simulink model "cpu_von_nuemann"  (R2020a)
settings: Solver=VariableStepAuto  StartTime=0.0  StopTime=10.0  RelTol=1e-3
libraries: simulink_extras x402, msbPllFoundation x1
(part 7 of 64)

== system cpu_von_nuemann/CPU/ALU/Multiplier/Subsystem7/Subsystem4 ==
  In1 : Inport
  In2 : Inport  Port=2
  In3 : Inport  Port=3
  In4 : Inport  Port=4
  In5 : Inport  Port=5
  In6 : Inport  Port=6
  In7 : Inport  Port=7
  In8 : Inport  Port=8
  In9 : Inport  Port=9
  In10 : Inport  Port=10
  In11 : Inport  Port=11
  In12 : Inport  Port=12
  In13 : Inport  Port=13
  In14 : Inport  Port=14
  In15 : Inport  Port=15
  In16 : Inport  Port=16
  Constant16 : Constant  Value=0
  Constant17 : Constant  Value=0
  Display{16..19} (4 alike) : Display
  Logical Operator : Logic  Operator=XOR  AllPortsSameDT=off  OutDataTypeStr=boolean
  Logical Operator1 : Logic  AllPortsSameDT=off  OutDataTypeStr=boolean
  Subsystem1 : Subsystem
  Subsystem15 : Subsystem
  Subsystem2 : Subsystem
  Subsystem3 : Subsystem
  Subsystem4 : Subsystem
  Subsystem5 : Subsystem
  Subsystem6 : Subsystem
  Out1 : Outport
  Out2 : Outport  Port=2
  Out3 : Outport  Port=3
  Out4 : Outport  Port=4
  Out5 : Outport  Port=5
  Out6 : Outport  Port=6
  Out7 : Outport  Port=7
  Out8 : Outport  Port=8
  Out9 : Outport  Port=9
  Out10 : Outport  Port=10
  Out11 : Outport  Port=11
  Out12 : Outport  Port=12
  Out13 : Outport  Port=13
  Out14 : Outport  Port=14
  Out15 : Outport  Port=15
  Out16 : Outport  Port=16
  wires:
  Subsystem3/9(Out9) -> Out16/1
  Subsystem2/6(Out6) -> Subsystem5/13(In13)
  Subsystem5/5(Out5) -> Subsystem4/4(In4)
  Subsystem1/4(Out4) -> Subsystem5/3(In3)
  Subsystem6/1(Out1) -> Display16/1
  Subsystem3/6(Out6) -> Out13/1
  Subsystem2/8(Out8) -> Subsystem5/15(In15)
  In6/1 -> Subsystem3/2(In2), Subsystem2/2(In2)
  Subsystem5/6(Out6) -> Subsystem4/5(In5)
  In4/1 -> Subsystem1/4(In4), Subsystem15/4(In4)
  Subsystem2/2(Out2) -> Subsystem5/9(In9)
  Subsystem2/5(Out5) -> Subsystem5/12(In12)
  Subsystem1/2(Out2) -> Subsystem5/1(In1)
  In2/1 -> Subsystem15/2(In2), Subsystem1/2(In2)
  Subsystem5/8(Out8) -> Subsystem4/7(In7)
  Logical Operator1/1 -> Subsystem6/11(In11)
  Subsystem15/2(Out2) -> Subsystem6/1(In1)
  Subsystem5/3(Out3) -> Subsystem4/2(In2)
  Subsystem2/3(Out3) -> Subsystem5/10(In10)
  Subsystem15/3(Out3) -> Subsystem6/2(In2)
  Constant17/1 -> Subsystem4/11(In11), Subsystem4/10(In10), Subsystem4/9(In9)
  In12/1 -> Subsystem2/8(In8), Subsystem15/8(In8)
  Subsystem4/3(Out3) -> Subsystem6/14(In14)
  Subsystem4/5(Out5) -> Subsystem6/16(In16)
  Subsystem1/6(Out6) -> Subsystem5/5(In5)
  Subsystem2/4(Out4) -> Subsystem5/11(In11)
  Subsystem15/5(Out5) -> Subsystem6/4(In4)
  Subsystem5/1(Out1) -> Logical Operator/1, Logical Operator1/2
  Subsystem1/8(Out8) -> Subsystem5/7(In7)
  Subsystem5/4(Out4) -> Subsystem4/3(In3)
  In8/1 -> Subsystem3/4(In4), Subsystem2/4(In4)
  In10/1 -> Subsystem2/6(In6), Subsystem15/6(In6)
  Subsystem5/2(Out2) -> Subsystem4/1(In1)
  Subsystem6/8(Out8) -> Out7/1
  Constant16/1 -> Subsystem6/10(In10), Subsystem6/9(In9)
  In9/1 -> Subsystem2/5(In5), Subsystem15/5(In5)
  Subsystem1/9(Out9) -> Subsystem5/8(In8)
  Subsystem3/1(Out1) -> Subsystem4/12(In12)
  Subsystem4/9(Out9) -> Out12/1
  In11/1 -> Subsystem2/7(In7), Subsystem15/7(In7)
  In1/1 -> Subsystem1/1(In1), Subsystem15/1(In1)
  In15/1 -> Subsystem3/7(In7), Subsystem1/7(In7)
  Subsystem5/7(Out7) -> Subsystem4/6(In6)
  Subsystem6/3(Out3) -> Out2/1
  In7/1 -> Subsystem3/3(In3), Subsystem2/3(In3)
  Subsystem15/6(Out6) -> Subsystem6/5(In5)
  Subsystem4/8(Out8) -> Out11/1
  Subsystem3/7(Out7) -> Out14/1
  Subsystem15/9(Out9) -> Subsystem6/8(In8)
  Subsystem15/8(Out8) -> Subsystem6/7(In7)
  Subsystem4/7(Out7) -> Out10/1
  Subsystem1/1(Out1) -> Display18/1
  Subsystem6/7(Out7) -> Out6/1
  In16/1 -> Subsystem3/8(In8), Subsystem1/8(In8)
  Subsystem6/4(Out4) -> Out3/1
  In5/1 -> Subsystem3/1(In1), Subsystem2/1(In1)
  Subsystem15/7(Out7) -> Subsystem6/6(In6)
  Subsystem15/4(Out4) -> Subsystem6/3(In3)
  In3/1 -> Subsystem15/3(In3), Subsystem1/3(In3)
  Subsystem3/5(Out5) -> Subsystem4/16(In16)
  Subsystem2/7(Out7) -> Subsystem5/14(In14)
  Logical Operator/1 -> Subsystem6/12(In12)
  Subsystem15/1(Out1) -> Display19/1
  Subsystem6/5(Out5) -> Out4/1
  Subsystem2/1(Out1) -> Display17/1
  Subsystem4/6(Out6) -> Out9/1
  Subsystem5/9(Out9) -> Subsystem4/8(In8)
  Subsystem4/1(Out1) -> Logical Operator/2, Logical Operator1/1
  Subsystem6/9(Out9) -> Out8/1
  Subsystem3/8(Out8) -> Out15/1
  Subsystem4/2(Out2) -> Subsystem6/13(In13)
  Subsystem3/2(Out2) -> Subsystem4/13(In13)
  Subsystem3/4(Out4) -> Subsystem4/15(In15)
  In13/1 -> Subsystem3/5(In5), Subsystem1/5(In5)
  Subsystem4/4(Out4) -> Subsystem6/15(In15)
  Subsystem6/6(Out6) -> Out5/1
  Subsystem2/9(Out9) -> Subsystem5/16(In16)
  Subsystem1/5(Out5) -> Subsystem5/4(In4)
  Subsystem3/3(Out3) -> Subsystem4/14(In14)
  Subsystem6/2(Out2) -> Out1/1
  Subsystem1/7(Out7) -> Subsystem5/6(In6)
  In14/1 -> Subsystem3/6(In6), Subsystem1/6(In6)
  Subsystem1/3(Out3) -> Subsystem5/2(In2)

== system cpu_von_nuemann/CPU/ALU/Multiplier/Subsystem7/Subsystem5 ==
  In1 : Inport
  In2 : Inport  Port=2
  In3 : Inport  Port=3
  In4 : Inport  Port=4
  In5 : Inport  Port=5
  In6 : Inport  Port=6
  In7 : Inport  Port=7
  In8 : Inport  Port=8
  In17 : Inport  Port=9
  In18 : Inport  Port=10
  In19 : Inport  Port=11
  In20 : Inport  Port=12
  14 : Inport  Port=13
  In22 : Inport  Port=14
  In23 : Inport  Port=15
  In24 : Inport  Port=16
  In9 : Inport  Port=17
  In10 : Inport  Port=18
  In11 : Inport  Port=19
  In12 : Inport  Port=20
  In13 : Inport  Port=21
  In14 : Inport  Port=22
  In15 : Inport  Port=23
  In16 : Inport  Port=24
  In25 : Inport  Port=25
  In26 : Inport  Port=26
  In27 : Inport  Port=27
  In28 : Inport  Port=28
  In29 : Inport  Port=29
  In30 : Inport  Port=30
  In31 : Inport  Port=31
  In32 : Inport  Port=32
  Subsystem5 : Subsystem
  Subsystem6 : Subsystem
  Out1 : Outport
  Out2 : Outport  Port=2
  Out3 : Outport  Port=3
  Out4 : Outport  Port=4
  Out5 : Outport  Port=5
  Out6 : Outport  Port=6
  Out7 : Outport  Port=7
  Out8 : Outport  Port=8
  Out9 : Outport  Port=9
  Out10 : Outport  Port=10
  Out11 : Outport  Port=11
  Out12 : Outport  Port=12
  Out13 : Outport  Port=13
  Out14 : Outport  Port=14
  Out15 : Outport  Port=15
  Out16 : Outport  Port=16
  Out17 : Outport  Port=17
  wires:
  In29/1 -> Subsystem6/13(In13)
  In15/1 -> Subsystem5/16(In15)
  In25/1 -> Subsystem6/9(In9)
  Subsystem6/3(Out3) -> Out11/1
  In30/1 -> Subsystem6/14(In14)
  Subsystem6/9(Out9) -> Out17/1
  In32/1 -> Subsystem6/16(In16)
  In18/1 -> Subsystem6/2(In2)
  Subsystem6/6(Out6) -> Out14/1
  In26/1 -> Subsystem6/10(In10)
  Subsystem5/4(Out4) -> Out4/1
  In24/1 -> Subsystem6/8(In8)
  Subsystem5/6(Out6) -> Out6/1
  Subsystem5/1(Out1) -> Out1/1
  In5/1 -> Subsystem5/5(In5)
  In1/1 -> Subsystem5/1(In1)
  In19/1 -> Subsystem6/3(In3)
  Subsystem6/5(Out5) -> Out13/1
  Subsystem5/8(Out8) -> Out8/1
  In28/1 -> Subsystem6/12(In12)
  In10/1 -> Subsystem5/11(In10)
  In14/1 -> Subsystem5/15(In14)
  Subsystem5/3(Out3) -> Out3/1
  In16/1 -> Subsystem5/17(In16)
  Subsystem5/2(Out2) -> Out2/1
  Subsystem5/9(Out9) -> Out9/1
  In8/1 -> Subsystem5/8(In8)
  Subsystem5/5(Out5) -> Out5/1
  In2/1 -> Subsystem5/2(In2)
  In17/1 -> Subsystem6/1(In1)
  In23/1 -> Subsystem6/7(In7)
  Subsystem6/4(Out4) -> Out12/1
  In27/1 -> Subsystem6/11(In11)
  In11/1 -> Subsystem5/12(In11)
  In13/1 -> Subsystem5/14(In13)
  Subsystem6/8(Out8) -> Out16/1
  In22/1 -> Subsystem6/6(In6)
  Subsystem6/1(Out1) -> Subsystem5/9(In17)
  In31/1 -> Subsystem6/15(In15)
  In7/1 -> Subsystem5/7(In7)
  In6/1 -> Subsystem5/6(In6)
  Subsystem6/7(Out7) -> Out15/1
  14/1 -> Subsystem6/5(In5)
  Subsystem6/2(Out2) -> Out10/1
  In4/1 -> Subsystem5/4(In4)
  In20/1 -> Subsystem6/4(In4)
  In12/1 -> Subsystem5/13(In12)
  In3/1 -> Subsystem5/3(In3)
  Subsystem5/7(Out7) -> Out7/1
  In9/1 -> Subsystem5/10(In9)

== system cpu_von_nuemann/CPU/ALU/Multiplier/Subsystem7/Subsystem6 ==
  In1 : Inport
  In2 : Inport  Port=2
  In3 : Inport  Port=3
  In4 : Inport  Port=4
  In5 : Inport  Port=5
  In6 : Inport  Port=6
  In7 : Inport  Port=7
  In8 : Inport  Port=8
  In17 : Inport  Port=9
  In18 : Inport  Port=10
  In19 : Inport  Port=11
  In20 : Inport  Port=12
  14 : Inport  Port=13
  In22 : Inport  Port=14
  In23 : Inport  Port=15
  In24 : Inport  Port=16
  In9 : Inport  Port=17
  In10 : Inport  Port=18
  In11 : Inport  Port=19
  In12 : Inport  Port=20
  In13 : Inport  Port=21
  In14 : Inport  Port=22
  In15 : Inport  Port=23
  In16 : Inport  Port=24
  In25 : Inport  Port=25
  In26 : Inport  Port=26
  In27 : Inport  Port=27
  In28 : Inport  Port=28
  In29 : Inport  Port=29
  In30 : Inport  Port=30
  In31 : Inport  Port=31
  In32 : Inport  Port=32
  Subsystem5 : Subsystem
  Subsystem6 : Subsystem
  Out1 : Outport
  Out2 : Outport  Port=2
  Out3 : Outport  Port=3
  Out4 : Outport  Port=4
  Out5 : Outport  Port=5
  Out6 : Outport  Port=6
  Out7 : Outport  Port=7
  Out8 : Outport  Port=8
  Out9 : Outport  Port=9
  Out10 : Outport  Port=10
  Out11 : Outport  Port=11
  Out12 : Outport  Port=12
  Out13 : Outport  Port=13
  Out14 : Outport  Port=14
  Out15 : Outport  Port=15
  Out16 : Outport  Port=16
  Out17 : Outport  Port=17
  wires:
  In29/1 -> Subsystem6/13(In13)
  In15/1 -> Subsystem5/16(In15)
  In25/1 -> Subsystem6/9(In9)
  Subsystem6/3(Out3) -> Out11/1
  In30/1 -> Subsystem6/14(In14)
  Subsystem6/9(Out9) -> Out17/1
  In32/1 -> Subsystem6/16(In16)
  In18/1 -> Subsystem6/2(In2)
  Subsystem6/6(Out6) -> Out14/1
  In26/1 -> Subsystem6/10(In10)
  Subsystem5/4(Out4) -> Out4/1
  In24/1 -> Subsystem6/8(In8)
  Subsystem5/6(Out6) -> Out6/1
  Subsystem5/1(Out1) -> Out1/1
  In5/1 -> Subsystem5/5(In5)
  In1/1 -> Subsystem5/1(In1)
  In19/1 -> Subsystem6/3(In3)
  Subsystem6/5(Out5) -> Out13/1
  Subsystem5/8(Out8) -> Out8/1
  In28/1 -> Subsystem6/12(In12)
  In10/1 -> Subsystem5/11(In10)
  In14/1 -> Subsystem5/15(In14)
  Subsystem5/3(Out3) -> Out3/1
  In16/1 -> Subsystem5/17(In16)
  Subsystem5/2(Out2) -> Out2/1
  Subsystem5/9(Out9) -> Out9/1
  In8/1 -> Subsystem5/8(In8)
  Subsystem5/5(Out5) -> Out5/1
  In2/1 -> Subsystem5/2(In2)
  In17/1 -> Subsystem6/1(In1)
  In23/1 -> Subsystem6/7(In7)
  Subsystem6/4(Out4) -> Out12/1
  In27/1 -> Subsystem6/11(In11)
  In11/1 -> Subsystem5/12(In11)
  In13/1 -> Subsystem5/14(In13)
  Subsystem6/8(Out8) -> Out16/1
  In22/1 -> Subsystem6/6(In6)
  Subsystem6/1(Out1) -> Subsystem5/9(In17)
  In31/1 -> Subsystem6/15(In15)
  In7/1 -> Subsystem5/7(In7)
  In6/1 -> Subsystem5/6(In6)
  Subsystem6/7(Out7) -> Out15/1
  14/1 -> Subsystem6/5(In5)
  Subsystem6/2(Out2) -> Out10/1
  In4/1 -> Subsystem5/4(In4)
  In20/1 -> Subsystem6/4(In4)
  In12/1 -> Subsystem5/13(In12)
  In3/1 -> Subsystem5/3(In3)
  Subsystem5/7(Out7) -> Out7/1
  In9/1 -> Subsystem5/10(In9)

== system cpu_von_nuemann/CPU/ALU/Subsystem7/Subsystem1/Subsystem1 ==
  In1 : Inport
  In2 : Inport  Port=2
  In3 : Inport  Port=3
  In4 : Inport  Port=4
  In5 : Inport  Port=5
  In7 : Inport  Port=6
  In6 : Inport  Port=7
  Demux{,1..3} (4 alike) : Demux  Outputs=8
  Mux : Mux  Inputs=8
  Subsystem : Subsystem
  Subsystem1 : Subsystem
  Subsystem2 : Subsystem
  Subsystem3 : Subsystem
  Subsystem4 : Subsystem
  Subsystem5 : Subsystem
  Subsystem6 : Subsystem
  Subsystem7 : Subsystem
  Out1 : Outport
  wires:
  Demux3/7 -> Subsystem6/6(In6)
  In6/1 -> Subsystem4/7(In7), Subsystem7/7(In7), Subsystem5/7(In7), Subsystem6/7(In7), Subsystem1/7(In7), Subsystem3/7(In7), Subsystem2/7(In7), Subsystem/7(In7)
  Subsystem3/1(Out1) -> Mux/4
  Demux/1 -> Subsystem/3(In3)
  Demux2/8 -> Subsystem7/5(In5)
  Subsystem1/1(Out1) -> Mux/2
  Subsystem2/1(Out1) -> Mux/3
  Subsystem4/1(Out1) -> Mux/5
  Demux1/2 -> Subsystem1/4(In4)
  Demux/6 -> Subsystem5/3(In3)
  In4/1 -> Demux1/1
  Demux2/7 -> Subsystem6/5(In5)
  In3/1 -> Demux/1
  Demux1/4 -> Subsystem3/4(In4)
  In2/1 -> Subsystem4/2(In2), Subsystem5/2(In2), Subsystem6/2(In2), Subsystem7/2(In2), Subsystem2/2(In2), Subsystem3/2(In2), Subsystem/2(In2), Subsystem1/2(In2)
  Demux3/3 -> Subsystem2/6(In6)
  Subsystem/1(Out1) -> Mux/1
  Subsystem5/1(Out1) -> Mux/6
  In7/1 -> Demux3/1
  Mux/1 -> Out1/1
  Demux/3 -> Subsystem2/3(In3)
  Demux1/8 -> Subsystem7/4(In4)
  Demux3/6 -> Subsystem5/6(In6)
  Demux3/1 -> Subsystem/6(In6)
  Demux3/2 -> Subsystem1/6(In6)
  Subsystem6/1(Out1) -> Mux/7
  Demux1/3 -> Subsystem2/4(In4)
  Demux2/4 -> Subsystem3/5(In5)
  Demux1/5 -> Subsystem4/4(In4)
  In1/1 -> Subsystem6/1(In1), Subsystem7/1(In1), Subsystem4/1(In1), Subsystem5/1(In1), Subsystem2/1(In1), Subsystem3/1(In1), Subsystem/1(In1), Subsystem1/1(In1)
  Demux1/1 -> Subsystem/4(In4)
  Demux3/4 -> Subsystem3/6(In6)
  Demux2/2 -> Subsystem1/5(In5)
  Demux2/6 -> Subsystem5/5(In5)
  Demux/2 -> Subsystem1/3(In3)
  Demux/7 -> Subsystem6/3(In3)
  Demux3/8 -> Subsystem7/6(In6)
  Demux1/6 -> Subsystem5/4(In4)
  Demux/5 -> Subsystem4/3(In3)
  Demux2/5 -> Subsystem4/5(In5)
  Demux/8 -> Subsystem7/3(In3)
  Demux2/3 -> Subsystem2/5(In5)
  Demux3/5 -> Subsystem4/6(In6)
  In5/1 -> Demux2/1
  Demux1/7 -> Subsystem6/4(In4)
  Subsystem7/1(Out1) -> Mux/8
  Demux/4 -> Subsystem3/3(In3)
  Demux2/1 -> Subsystem/5(In5)

== system cpu_von_nuemann/CPU/ALU/Subsystem7/Subsystem1/Subsystem2 ==
  In1 : Inport
  In2 : Inport  Port=2
  In3 : Inport  Port=3
  In4 : Inport  Port=4
  In5 : Inport  Port=5
  In7 : Inport  Port=6
  In6 : Inport  Port=7
  Demux{,1..3} (4 alike) : Demux  Outputs=8
  Mux : Mux  Inputs=8
  Subsystem : Subsystem
  Subsystem1 : Subsystem
  Subsystem2 : Subsystem
  Subsystem3 : Subsystem
  Subsystem4 : Subsystem
  Subsystem5 : Subsystem
  Subsystem6 : Subsystem
  Subsystem7 : Subsystem
  Out1 : Outport
  wires:
  Demux3/7 -> Subsystem6/6(In6)
  In6/1 -> Subsystem4/7(In7), Subsystem7/7(In7), Subsystem5/7(In7), Subsystem6/7(In7), Subsystem1/7(In7), Subsystem3/7(In7), Subsystem2/7(In7), Subsystem/7(In7)
  Subsystem3/1(Out1) -> Mux/4
  Demux/1 -> Subsystem/3(In3)
  Demux2/8 -> Subsystem7/5(In5)
  Subsystem1/1(Out1) -> Mux/2
  Subsystem2/1(Out1) -> Mux/3
  Subsystem4/1(Out1) -> Mux/5
  Demux1/2 -> Subsystem1/4(In4)
  Demux/6 -> Subsystem5/3(In3)
  In4/1 -> Demux1/1
  Demux2/7 -> Subsystem6/5(In5)
  In3/1 -> Demux/1
  Demux1/4 -> Subsystem3/4(In4)
  In2/1 -> Subsystem4/2(In2), Subsystem5/2(In2), Subsystem6/2(In2), Subsystem7/2(In2), Subsystem2/2(In2), Subsystem3/2(In2), Subsystem/2(In2), Subsystem1/2(In2)
  Demux3/3 -> Subsystem2/6(In6)
  Subsystem/1(Out1) -> Mux/1
  Subsystem5/1(Out1) -> Mux/6
  In7/1 -> Demux3/1
  Mux/1 -> Out1/1
  Demux/3 -> Subsystem2/3(In3)
  Demux1/8 -> Subsystem7/4(In4)
  Demux3/6 -> Subsystem5/6(In6)
  Demux3/1 -> Subsystem/6(In6)
  Demux3/2 -> Subsystem1/6(In6)
  Subsystem6/1(Out1) -> Mux/7
  Demux1/3 -> Subsystem2/4(In4)
  Demux2/4 -> Subsystem3/5(In5)
  Demux1/5 -> Subsystem4/4(In4)
  In1/1 -> Subsystem6/1(In1), Subsystem7/1(In1), Subsystem4/1(In1), Subsystem5/1(In1), Subsystem2/1(In1), Subsystem3/1(In1), Subsystem/1(In1), Subsystem1/1(In1)
  Demux1/1 -> Subsystem/4(In4)
  Demux3/4 -> Subsystem3/6(In6)
  Demux2/2 -> Subsystem1/5(In5)
  Demux2/6 -> Subsystem5/5(In5)
  Demux/2 -> Subsystem1/3(In3)
  Demux/7 -> Subsystem6/3(In3)
  Demux3/8 -> Subsystem7/6(In6)
  Demux1/6 -> Subsystem5/4(In4)
  Demux/5 -> Subsystem4/3(In3)
  Demux2/5 -> Subsystem4/5(In5)
  Demux/8 -> Subsystem7/3(In3)
  Demux2/3 -> Subsystem2/5(In5)
  Demux3/5 -> Subsystem4/6(In6)
  In5/1 -> Demux2/1
  Demux1/7 -> Subsystem6/4(In4)
  Subsystem7/1(Out1) -> Mux/8
  Demux/4 -> Subsystem3/3(In3)
  Demux2/1 -> Subsystem/5(In5)

== system cpu_von_nuemann/CPU/ALU/Subsystem7/Subsystem1/Subsystem3 ==
  In1 : Inport
  In2 : Inport  Port=2
  In3 : Inport  Port=3
  In4 : Inport  Port=4
  In5 : Inport  Port=5
  In7 : Inport  Port=6
  In6 : Inport  Port=7
  Demux{,1..3} (4 alike) : Demux  Outputs=8
  Mux : Mux  Inputs=8
  Subsystem : Subsystem
  Subsystem1 : Subsystem
  Subsystem2 : Subsystem
  Subsystem3 : Subsystem
  Subsystem4 : Subsystem
  Subsystem5 : Subsystem
  Subsystem6 : Subsystem
  Subsystem7 : Subsystem
  Out1 : Outport
  wires:
  Demux3/7 -> Subsystem6/6(In6)
  In6/1 -> Subsystem4/7(In7), Subsystem7/7(In7), Subsystem5/7(In7), Subsystem6/7(In7), Subsystem1/7(In7), Subsystem3/7(In7), Subsystem2/7(In7), Subsystem/7(In7)
  Subsystem3/1(Out1) -> Mux/4
  Demux/1 -> Subsystem/3(In3)
  Demux2/8 -> Subsystem7/5(In5)
  Subsystem1/1(Out1) -> Mux/2
  Subsystem2/1(Out1) -> Mux/3
  Subsystem4/1(Out1) -> Mux/5
  Demux1/2 -> Subsystem1/4(In4)
  Demux/6 -> Subsystem5/3(In3)
  In4/1 -> Demux1/1
  Demux2/7 -> Subsystem6/5(In5)
  In3/1 -> Demux/1
  Demux1/4 -> Subsystem3/4(In4)
  In2/1 -> Subsystem4/2(In2), Subsystem5/2(In2), Subsystem6/2(In2), Subsystem7/2(In2), Subsystem2/2(In2), Subsystem3/2(In2), Subsystem/2(In2), Subsystem1/2(In2)
  Demux3/3 -> Subsystem2/6(In6)
  Subsystem/1(Out1) -> Mux/1
  Subsystem5/1(Out1) -> Mux/6
  In7/1 -> Demux3/1
  Mux/1 -> Out1/1
  Demux/3 -> Subsystem2/3(In3)
  Demux1/8 -> Subsystem7/4(In4)
  Demux3/6 -> Subsystem5/6(In6)
  Demux3/1 -> Subsystem/6(In6)
  Demux3/2 -> Subsystem1/6(In6)
  Subsystem6/1(Out1) -> Mux/7
  Demux1/3 -> Subsystem2/4(In4)
  Demux2/4 -> Subsystem3/5(In5)
  Demux1/5 -> Subsystem4/4(In4)
  In1/1 -> Subsystem6/1(In1), Subsystem7/1(In1), Subsystem4/1(In1), Subsystem5/1(In1), Subsystem2/1(In1), Subsystem3/1(In1), Subsystem/1(In1), Subsystem1/1(In1)
  Demux1/1 -> Subsystem/4(In4)
  Demux3/4 -> Subsystem3/6(In6)
  Demux2/2 -> Subsystem1/5(In5)
  Demux2/6 -> Subsystem5/5(In5)
  Demux/2 -> Subsystem1/3(In3)
  Demux/7 -> Subsystem6/3(In3)
  Demux3/8 -> Subsystem7/6(In6)
  Demux1/6 -> Subsystem5/4(In4)
  Demux/5 -> Subsystem4/3(In3)
  Demux2/5 -> Subsystem4/5(In5)
  Demux/8 -> Subsystem7/3(In3)
  Demux2/3 -> Subsystem2/5(In5)
  Demux3/5 -> Subsystem4/6(In6)
  In5/1 -> Demux2/1
  Demux1/7 -> Subsystem6/4(In4)
  Subsystem7/1(Out1) -> Mux/8
  Demux/4 -> Subsystem3/3(In3)
  Demux2/1 -> Subsystem/5(In5)

== system cpu_von_nuemann/CPU/ALU/Subsystem7/Subsystem1/Subsystem4 ==
  In1 : Inport
  In2 : Inport  Port=2
  In3 : Inport  Port=3
  In4 : Inport  Port=4
  In5 : Inport  Port=5
  In7 : Inport  Port=6
  In6 : Inport  Port=7
  Demux{,1..3} (4 alike) : Demux  Outputs=8
  Mux : Mux  Inputs=8
  Subsystem : Subsystem
  Subsystem1 : Subsystem
  Subsystem2 : Subsystem
  Subsystem3 : Subsystem
  Subsystem4 : Subsystem
  Subsystem5 : Subsystem
  Subsystem6 : Subsystem
  Subsystem7 : Subsystem
  Out1 : Outport
  wires:
  Demux3/7 -> Subsystem6/6(In6)
  In6/1 -> Subsystem4/7(In7), Subsystem7/7(In7), Subsystem5/7(In7), Subsystem6/7(In7), Subsystem1/7(In7), Subsystem3/7(In7), Subsystem2/7(In7), Subsystem/7(In7)
  Subsystem3/1(Out1) -> Mux/4
  Demux/1 -> Subsystem/3(In3)
  Demux2/8 -> Subsystem7/5(In5)
  Subsystem1/1(Out1) -> Mux/2
  Subsystem2/1(Out1) -> Mux/3
  Subsystem4/1(Out1) -> Mux/5
  Demux1/2 -> Subsystem1/4(In4)
  Demux/6 -> Subsystem5/3(In3)
  In4/1 -> Demux1/1
  Demux2/7 -> Subsystem6/5(In5)
  In3/1 -> Demux/1
  Demux1/4 -> Subsystem3/4(In4)
  In2/1 -> Subsystem4/2(In2), Subsystem5/2(In2), Subsystem6/2(In2), Subsystem7/2(In2), Subsystem2/2(In2), Subsystem3/2(In2), Subsystem/2(In2), Subsystem1/2(In2)
  Demux3/3 -> Subsystem2/6(In6)
  Subsystem/1(Out1) -> Mux/1
  Subsystem5/1(Out1) -> Mux/6
  In7/1 -> Demux3/1
  Mux/1 -> Out1/1
  Demux/3 -> Subsystem2/3(In3)
  Demux1/8 -> Subsystem7/4(In4)
  Demux3/6 -> Subsystem5/6(In6)
  Demux3/1 -> Subsystem/6(In6)
  Demux3/2 -> Subsystem1/6(In6)
  Subsystem6/1(Out1) -> Mux/7
  Demux1/3 -> Subsystem2/4(In4)
  Demux2/4 -> Subsystem3/5(In5)
  Demux1/5 -> Subsystem4/4(In4)
  In1/1 -> Subsystem6/1(In1), Subsystem7/1(In1), Subsystem4/1(In1), Subsystem5/1(In1), Subsystem2/1(In1), Subsystem3/1(In1), Subsystem/1(In1), Subsystem1/1(In1)
  Demux1/1 -> Subsystem/4(In4)
  Demux3/4 -> Subsystem3/6(In6)
  Demux2/2 -> Subsystem1/5(In5)
  Demux2/6 -> Subsystem5/5(In5)
  Demux/2 -> Subsystem1/3(In3)
  Demux/7 -> Subsystem6/3(In3)
  Demux3/8 -> Subsystem7/6(In6)
  Demux1/6 -> Subsystem5/4(In4)
  Demux/5 -> Subsystem4/3(In3)
  Demux2/5 -> Subsystem4/5(In5)
  Demux/8 -> Subsystem7/3(In3)
  Demux2/3 -> Subsystem2/5(In5)
  Demux3/5 -> Subsystem4/6(In6)
  In5/1 -> Demux2/1
  Demux1/7 -> Subsystem6/4(In4)
  Subsystem7/1(Out1) -> Mux/8
  Demux/4 -> Subsystem3/3(In3)
  Demux2/1 -> Subsystem/5(In5)

== system cpu_von_nuemann/CPU/ALU/Subsystem7/Subsystem1/Subsystem5 ==
  In1 : Inport
  In2 : Inport  Port=2
  In3 : Inport  Port=3
  In4 : Inport  Port=4
  In5 : Inport  Port=5
  In7 : Inport  Port=6
  In6 : Inport  Port=7
  Demux{,1..3} (4 alike) : Demux  Outputs=8
  Mux : Mux  Inputs=8
  Subsystem : Subsystem
  Subsystem1 : Subsystem
  Subsystem2 : Subsystem
  Subsystem3 : Subsystem
  Subsystem4 : Subsystem
  Subsystem5 : Subsystem
  Subsystem6 : Subsystem
  Subsystem7 : Subsystem
  Out1 : Outport
  wires:
  Demux3/7 -> Subsystem6/6(In6)
  In6/1 -> Subsystem4/7(In7), Subsystem7/7(In7), Subsystem5/7(In7), Subsystem6/7(In7), Subsystem1/7(In7), Subsystem3/7(In7), Subsystem2/7(In7), Subsystem/7(In7)
  Subsystem3/1(Out1) -> Mux/4
  Demux/1 -> Subsystem/3(In3)
  Demux2/8 -> Subsystem7/5(In5)
  Subsystem1/1(Out1) -> Mux/2
  Subsystem2/1(Out1) -> Mux/3
  Subsystem4/1(Out1) -> Mux/5
  Demux1/2 -> Subsystem1/4(In4)
  Demux/6 -> Subsystem5/3(In3)
  In4/1 -> Demux1/1
  Demux2/7 -> Subsystem6/5(In5)
  In3/1 -> Demux/1
  Demux1/4 -> Subsystem3/4(In4)
  In2/1 -> Subsystem4/2(In2), Subsystem5/2(In2), Subsystem6/2(In2), Subsystem7/2(In2), Subsystem2/2(In2), Subsystem3/2(In2), Subsystem/2(In2), Subsystem1/2(In2)
  Demux3/3 -> Subsystem2/6(In6)
  Subsystem/1(Out1) -> Mux/1
  Subsystem5/1(Out1) -> Mux/6
  In7/1 -> Demux3/1
  Mux/1 -> Out1/1
  Demux/3 -> Subsystem2/3(In3)
  Demux1/8 -> Subsystem7/4(In4)
  Demux3/6 -> Subsystem5/6(In6)
  Demux3/1 -> Subsystem/6(In6)
  Demux3/2 -> Subsystem1/6(In6)
  Subsystem6/1(Out1) -> Mux/7
  Demux1/3 -> Subsystem2/4(In4)
  Demux2/4 -> Subsystem3/5(In5)
  Demux1/5 -> Subsystem4/4(In4)
  In1/1 -> Subsystem6/1(In1), Subsystem7/1(In1), Subsystem4/1(In1), Subsystem5/1(In1), Subsystem2/1(In1), Subsystem3/1(In1), Subsystem/1(In1), Subsystem1/1(In1)
  Demux1/1 -> Subsystem/4(In4)
  Demux3/4 -> Subsystem3/6(In6)
  Demux2/2 -> Subsystem1/5(In5)
  Demux2/6 -> Subsystem5/5(In5)
  Demux/2 -> Subsystem1/3(In3)
  Demux/7 -> Subsystem6/3(In3)
  Demux3/8 -> Subsystem7/6(In6)
  Demux1/6 -> Subsystem5/4(In4)
  Demux/5 -> Subsystem4/3(In3)
  Demux2/5 -> Subsystem4/5(In5)
  Demux/8 -> Subsystem7/3(In3)
  Demux2/3 -> Subsystem2/5(In5)
  Demux3/5 -> Subsystem4/6(In6)
  In5/1 -> Demux2/1
  Demux1/7 -> Subsystem6/4(In4)
  Subsystem7/1(Out1) -> Mux/8
  Demux/4 -> Subsystem3/3(In3)
  Demux2/1 -> Subsystem/5(In5)

== system cpu_von_nuemann/CPU/ALU/Subsystem7/Subsystem2/Subsystem1 ==
  In1 : Inport
  In2 : Inport  Port=2
  In3 : Inport  Port=3
  In4 : Inport  Port=4
  In5 : Inport  Port=5
  In7 : Inport  Port=6
  In6 : Inport  Port=7
  Demux{,1..3} (4 alike) : Demux  Outputs=8
  Mux : Mux  Inputs=8
  Subsystem : Subsystem
  Subsystem1 : Subsystem
  Subsystem2 : Subsystem
  Subsystem3 : Subsystem
  Subsystem4 : Subsystem
  Subsystem5 : Subsystem
  Subsystem6 : Subsystem
  Subsystem7 : Subsystem
  Out1 : Outport
  wires:
  Demux3/7 -> Subsystem6/6(In6)
  In6/1 -> Subsystem4/7(In7), Subsystem7/7(In7), Subsystem5/7(In7), Subsystem6/7(In7), Subsystem1/7(In7), Subsystem3/7(In7), Subsystem2/7(In7), Subsystem/7(In7)
  Subsystem3/1(Out1) -> Mux/4
  Demux/1 -> Subsystem/3(In3)
  Demux2/8 -> Subsystem7/5(In5)
  Subsystem1/1(Out1) -> Mux/2
  Subsystem2/1(Out1) -> Mux/3
  Subsystem4/1(Out1) -> Mux/5
  Demux1/2 -> Subsystem1/4(In4)
  Demux/6 -> Subsystem5/3(In3)
  In4/1 -> Demux1/1
  Demux2/7 -> Subsystem6/5(In5)
  In3/1 -> Demux/1
  Demux1/4 -> Subsystem3/4(In4)
  In2/1 -> Subsystem4/2(In2), Subsystem5/2(In2), Subsystem6/2(In2), Subsystem7/2(In2), Subsystem2/2(In2), Subsystem3/2(In2), Subsystem/2(In2), Subsystem1/2(In2)
  Demux3/3 -> Subsystem2/6(In6)
  Subsystem/1(Out1) -> Mux/1
  Subsystem5/1(Out1) -> Mux/6
  In7/1 -> Demux3/1
  Mux/1 -> Out1/1
  Demux/3 -> Subsystem2/3(In3)
  Demux1/8 -> Subsystem7/4(In4)
  Demux3/6 -> Subsystem5/6(In6)
  Demux3/1 -> Subsystem/6(In6)
  Demux3/2 -> Subsystem1/6(In6)
  Subsystem6/1(Out1) -> Mux/7
  Demux1/3 -> Subsystem2/4(In4)
  Demux2/4 -> Subsystem3/5(In5)
  Demux1/5 -> Subsystem4/4(In4)
  In1/1 -> Subsystem6/1(In1), Subsystem7/1(In1), Subsystem4/1(In1), Subsystem5/1(In1), Subsystem2/1(In1), Subsystem3/1(In1), Subsystem/1(In1), Subsystem1/1(In1)
  Demux1/1 -> Subsystem/4(In4)
  Demux3/4 -> Subsystem3/6(In6)
  Demux2/2 -> Subsystem1/5(In5)
  Demux2/6 -> Subsystem5/5(In5)
  Demux/2 -> Subsystem1/3(In3)
  Demux/7 -> Subsystem6/3(In3)
  Demux3/8 -> Subsystem7/6(In6)
  Demux1/6 -> Subsystem5/4(In4)
  Demux/5 -> Subsystem4/3(In3)
  Demux2/5 -> Subsystem4/5(In5)
  Demux/8 -> Subsystem7/3(In3)
  Demux2/3 -> Subsystem2/5(In5)
  Demux3/5 -> Subsystem4/6(In6)
  In5/1 -> Demux2/1
  Demux1/7 -> Subsystem6/4(In4)
  Subsystem7/1(Out1) -> Mux/8
  Demux/4 -> Subsystem3/3(In3)
  Demux2/1 -> Subsystem/5(In5)

== system cpu_von_nuemann/CPU/ALU/Subsystem7/Subsystem2/Subsystem2 ==
  In1 : Inport
  In2 : Inport  Port=2
  In3 : Inport  Port=3
  In4 : Inport  Port=4
  In5 : Inport  Port=5
  In7 : Inport  Port=6
  In6 : Inport  Port=7
  Demux{,1..3} (4 alike) : Demux  Outputs=8
  Mux : Mux  Inputs=8
  Subsystem : Subsystem
  Subsystem1 : Subsystem
  Subsystem2 : Subsystem
  Subsystem3 : Subsystem
  Subsystem4 : Subsystem
  Subsystem5 : Subsystem
  Subsystem6 : Subsystem
  Subsystem7 : Subsystem
  Out1 : Outport
  wires:
  Demux3/7 -> Subsystem6/6(In6)
  In6/1 -> Subsystem4/7(In7), Subsystem7/7(In7), Subsystem5/7(In7), Subsystem6/7(In7), Subsystem1/7(In7), Subsystem3/7(In7), Subsystem2/7(In7), Subsystem/7(In7)
  Subsystem3/1(Out1) -> Mux/4
  Demux/1 -> Subsystem/3(In3)
  Demux2/8 -> Subsystem7/5(In5)
  Subsystem1/1(Out1) -> Mux/2
  Subsystem2/1(Out1) -> Mux/3
  Subsystem4/1(Out1) -> Mux/5
  Demux1/2 -> Subsystem1/4(In4)
  Demux/6 -> Subsystem5/3(In3)
  In4/1 -> Demux1/1
  Demux2/7 -> Subsystem6/5(In5)
  In3/1 -> Demux/1
  Demux1/4 -> Subsystem3/4(In4)
  In2/1 -> Subsystem4/2(In2), Subsystem5/2(In2), Subsystem6/2(In2), Subsystem7/2(In2), Subsystem2/2(In2), Subsystem3/2(In2), Subsystem/2(In2), Subsystem1/2(In2)
  Demux3/3 -> Subsystem2/6(In6)
  Subsystem/1(Out1) -> Mux/1
  Subsystem5/1(Out1) -> Mux/6
  In7/1 -> Demux3/1
  Mux/1 -> Out1/1
  Demux/3 -> Subsystem2/3(In3)
  Demux1/8 -> Subsystem7/4(In4)
  Demux3/6 -> Subsystem5/6(In6)
  Demux3/1 -> Subsystem/6(In6)
  Demux3/2 -> Subsystem1/6(In6)
  Subsystem6/1(Out1) -> Mux/7
  Demux1/3 -> Subsystem2/4(In4)
  Demux2/4 -> Subsystem3/5(In5)
  Demux1/5 -> Subsystem4/4(In4)
  In1/1 -> Subsystem6/1(In1), Subsystem7/1(In1), Subsystem4/1(In1), Subsystem5/1(In1), Subsystem2/1(In1), Subsystem3/1(In1), Subsystem/1(In1), Subsystem1/1(In1)
  Demux1/1 -> Subsystem/4(In4)
  Demux3/4 -> Subsystem3/6(In6)
  Demux2/2 -> Subsystem1/5(In5)
  Demux2/6 -> Subsystem5/5(In5)
  Demux/2 -> Subsystem1/3(In3)
  Demux/7 -> Subsystem6/3(In3)
  Demux3/8 -> Subsystem7/6(In6)
  Demux1/6 -> Subsystem5/4(In4)
  Demux/5 -> Subsystem4/3(In3)
  Demux2/5 -> Subsystem4/5(In5)
  Demux/8 -> Subsystem7/3(In3)
  Demux2/3 -> Subsystem2/5(In5)
  Demux3/5 -> Subsystem4/6(In6)
  In5/1 -> Demux2/1
  Demux1/7 -> Subsystem6/4(In4)
  Subsystem7/1(Out1) -> Mux/8
  Demux/4 -> Subsystem3/3(In3)
  Demux2/1 -> Subsystem/5(In5)

== system cpu_von_nuemann/CPU/ALU/Subsystem7/Subsystem2/Subsystem3 ==
  In1 : Inport
  In2 : Inport  Port=2
  In3 : Inport  Port=3
  In4 : Inport  Port=4
  In5 : Inport  Port=5
  In7 : Inport  Port=6
  In6 : Inport  Port=7
  Demux{,1..3} (4 alike) : Demux  Outputs=8
  Mux : Mux  Inputs=8
  Subsystem : Subsystem
  Subsystem1 : Subsystem
  Subsystem2 : Subsystem
  Subsystem3 : Subsystem
  Subsystem4 : Subsystem
  Subsystem5 : Subsystem
  Subsystem6 : Subsystem
  Subsystem7 : Subsystem
  Out1 : Outport
  wires:
  Demux3/7 -> Subsystem6/6(In6)
  In6/1 -> Subsystem4/7(In7), Subsystem7/7(In7), Subsystem5/7(In7), Subsystem6/7(In7), Subsystem1/7(In7), Subsystem3/7(In7), Subsystem2/7(In7), Subsystem/7(In7)
  Subsystem3/1(Out1) -> Mux/4
  Demux/1 -> Subsystem/3(In3)
  Demux2/8 -> Subsystem7/5(In5)
  Subsystem1/1(Out1) -> Mux/2
  Subsystem2/1(Out1) -> Mux/3
  Subsystem4/1(Out1) -> Mux/5
  Demux1/2 -> Subsystem1/4(In4)
  Demux/6 -> Subsystem5/3(In3)
  In4/1 -> Demux1/1
  Demux2/7 -> Subsystem6/5(In5)
  In3/1 -> Demux/1
  Demux1/4 -> Subsystem3/4(In4)
  In2/1 -> Subsystem4/2(In2), Subsystem5/2(In2), Subsystem6/2(In2), Subsystem7/2(In2), Subsystem2/2(In2), Subsystem3/2(In2), Subsystem/2(In2), Subsystem1/2(In2)
  Demux3/3 -> Subsystem2/6(In6)
  Subsystem/1(Out1) -> Mux/1
  Subsystem5/1(Out1) -> Mux/6
  In7/1 -> Demux3/1
  Mux/1 -> Out1/1
  Demux/3 -> Subsystem2/3(In3)
  Demux1/8 -> Subsystem7/4(In4)
  Demux3/6 -> Subsystem5/6(In6)
  Demux3/1 -> Subsystem/6(In6)
  Demux3/2 -> Subsystem1/6(In6)
  Subsystem6/1(Out1) -> Mux/7
  Demux1/3 -> Subsystem2/4(In4)
  Demux2/4 -> Subsystem3/5(In5)
  Demux1/5 -> Subsystem4/4(In4)
  In1/1 -> Subsystem6/1(In1), Subsystem7/1(In1), Subsystem4/1(In1), Subsystem5/1(In1), Subsystem2/1(In1), Subsystem3/1(In1), Subsystem/1(In1), Subsystem1/1(In1)
  Demux1/1 -> Subsystem/4(In4)
  Demux3/4 -> Subsystem3/6(In6)
  Demux2/2 -> Subsystem1/5(In5)
  Demux2/6 -> Subsystem5/5(In5)
  Demux/2 -> Subsystem1/3(In3)
  Demux/7 -> Subsystem6/3(In3)
  Demux3/8 -> Subsystem7/6(In6)
  Demux1/6 -> Subsystem5/4(In4)
  Demux/5 -> Subsystem4/3(In3)
  Demux2/5 -> Subsystem4/5(In5)
  Demux/8 -> Subsystem7/3(In3)
  Demux2/3 -> Subsystem2/5(In5)
  Demux3/5 -> Subsystem4/6(In6)
  In5/1 -> Demux2/1
  Demux1/7 -> Subsystem6/4(In4)
  Subsystem7/1(Out1) -> Mux/8
  Demux/4 -> Subsystem3/3(In3)
  Demux2/1 -> Subsystem/5(In5)

== system cpu_von_nuemann/CPU/ALU/Subsystem7/Subsystem2/Subsystem4 ==
  In1 : Inport
  In2 : Inport  Port=2
  In3 : Inport  Port=3
  In4 : Inport  Port=4
  In5 : Inport  Port=5
  In7 : Inport  Port=6
  In6 : Inport  Port=7
  Demux{,1..3} (4 alike) : Demux  Outputs=8
  Mux : Mux  Inputs=8
  Subsystem : Subsystem
  Subsystem1 : Subsystem
  Subsystem2 : Subsystem
  Subsystem3 : Subsystem
  Subsystem4 : Subsystem
  Subsystem5 : Subsystem
  Subsystem6 : Subsystem
  Subsystem7 : Subsystem
  Out1 : Outport
  wires:
  Demux3/7 -> Subsystem6/6(In6)
  In6/1 -> Subsystem4/7(In7), Subsystem7/7(In7), Subsystem5/7(In7), Subsystem6/7(In7), Subsystem1/7(In7), Subsystem3/7(In7), Subsystem2/7(In7), Subsystem/7(In7)
  Subsystem3/1(Out1) -> Mux/4
  Demux/1 -> Subsystem/3(In3)
  Demux2/8 -> Subsystem7/5(In5)
  Subsystem1/1(Out1) -> Mux/2
  Subsystem2/1(Out1) -> Mux/3
  Subsystem4/1(Out1) -> Mux/5
  Demux1/2 -> Subsystem1/4(In4)
  Demux/6 -> Subsystem5/3(In3)
  In4/1 -> Demux1/1
  Demux2/7 -> Subsystem6/5(In5)
  In3/1 -> Demux/1
  Demux1/4 -> Subsystem3/4(In4)
  In2/1 -> Subsystem4/2(In2), Subsystem5/2(In2), Subsystem6/2(In2), Subsystem7/2(In2), Subsystem2/2(In2), Subsystem3/2(In2), Subsystem/2(In2), Subsystem1/2(In2)
  Demux3/3 -> Subsystem2/6(In6)
  Subsystem/1(Out1) -> Mux/1
  Subsystem5/1(Out1) -> Mux/6
  In7/1 -> Demux3/1
  Mux/1 -> Out1/1
  Demux/3 -> Subsystem2/3(In3)
  Demux1/8 -> Subsystem7/4(In4)
  Demux3/6 -> Subsystem5/6(In6)
  Demux3/1 -> Subsystem/6(In6)
  Demux3/2 -> Subsystem1/6(In6)
  Subsystem6/1(Out1) -> Mux/7
  Demux1/3 -> Subsystem2/4(In4)
  Demux2/4 -> Subsystem3/5(In5)
  Demux1/5 -> Subsystem4/4(In4)
  In1/1 -> Subsystem6/1(In1), Subsystem7/1(In1), Subsystem4/1(In1), Subsystem5/1(In1), Subsystem2/1(In1), Subsystem3/1(In1), Subsystem/1(In1), Subsystem1/1(In1)
  Demux1/1 -> Subsystem/4(In4)
  Demux3/4 -> Subsystem3/6(In6)
  Demux2/2 -> Subsystem1/5(In5)
  Demux2/6 -> Subsystem5/5(In5)
  Demux/2 -> Subsystem1/3(In3)
  Demux/7 -> Subsystem6/3(In3)
  Demux3/8 -> Subsystem7/6(In6)
  Demux1/6 -> Subsystem5/4(In4)
  Demux/5 -> Subsystem4/3(In3)
  Demux2/5 -> Subsystem4/5(In5)
  Demux/8 -> Subsystem7/3(In3)
  Demux2/3 -> Subsystem2/5(In5)
  Demux3/5 -> Subsystem4/6(In6)
  In5/1 -> Demux2/1
  Demux1/7 -> Subsystem6/4(In4)
  Subsystem7/1(Out1) -> Mux/8
  Demux/4 -> Subsystem3/3(In3)
  Demux2/1 -> Subsystem/5(In5)

== system cpu_von_nuemann/CPU/ALU/Subsystem7/Subsystem2/Subsystem5 ==
  In1 : Inport
  In2 : Inport  Port=2
  In3 : Inport  Port=3
  In4 : Inport  Port=4
  In5 : Inport  Port=5
  In7 : Inport  Port=6
  In6 : Inport  Port=7
  Demux{,1..3} (4 alike) : Demux  Outputs=8
  Mux : Mux  Inputs=8
  Subsystem : Subsystem
  Subsystem1 : Subsystem
  Subsystem2 : Subsystem
  Subsystem3 : Subsystem
  Subsystem4 : Subsystem
  Subsystem5 : Subsystem
  Subsystem6 : Subsystem
  Subsystem7 : Subsystem
  Out1 : Outport
  wires:
  Demux3/7 -> Subsystem6/6(In6)
  In6/1 -> Subsystem4/7(In7), Subsystem7/7(In7), Subsystem5/7(In7), Subsystem6/7(In7), Subsystem1/7(In7), Subsystem3/7(In7), Subsystem2/7(In7), Subsystem/7(In7)
  Subsystem3/1(Out1) -> Mux/4
  Demux/1 -> Subsystem/3(In3)
  Demux2/8 -> Subsystem7/5(In5)
  Subsystem1/1(Out1) -> Mux/2
  Subsystem2/1(Out1) -> Mux/3
  Subsystem4/1(Out1) -> Mux/5
  Demux1/2 -> Subsystem1/4(In4)
  Demux/6 -> Subsystem5/3(In3)
  In4/1 -> Demux1/1
  Demux2/7 -> Subsystem6/5(In5)
  In3/1 -> Demux/1
  Demux1/4 -> Subsystem3/4(In4)
  In2/1 -> Subsystem4/2(In2), Subsystem5/2(In2), Subsystem6/2(In2), Subsystem7/2(In2), Subsystem2/2(In2), Subsystem3/2(In2), Subsystem/2(In2), Subsystem1/2(In2)
  Demux3/3 -> Subsystem2/6(In6)
  Subsystem/1(Out1) -> Mux/1
  Subsystem5/1(Out1) -> Mux/6
  In7/1 -> Demux3/1
  Mux/1 -> Out1/1
  Demux/3 -> Subsystem2/3(In3)
  Demux1/8 -> Subsystem7/4(In4)
  Demux3/6 -> Subsystem5/6(In6)
  Demux3/1 -> Subsystem/6(In6)
  Demux3/2 -> Subsystem1/6(In6)
  Subsystem6/1(Out1) -> Mux/7
  Demux1/3 -> Subsystem2/4(In4)
  Demux2/4 -> Subsystem3/5(In5)
  Demux1/5 -> Subsystem4/4(In4)
  In1/1 -> Subsystem6/1(In1), Subsystem7/1(In1), Subsystem4/1(In1), Subsystem5/1(In1), Subsystem2/1(In1), Subsystem3/1(In1), Subsystem/1(In1), Subsystem1/1(In1)
  Demux1/1 -> Subsystem/4(In4)
  Demux3/4 -> Subsystem3/6(In6)
  Demux2/2 -> Subsystem1/5(In5)
  Demux2/6 -> Subsystem5/5(In5)
  Demux/2 -> Subsystem1/3(In3)
  Demux/7 -> Subsystem6/3(In3)
  Demux3/8 -> Subsystem7/6(In6)
  Demux1/6 -> Subsystem5/4(In4)
  Demux/5 -> Subsystem4/3(In3)
  Demux2/5 -> Subsystem4/5(In5)
  Demux/8 -> Subsystem7/3(In3)
  Demux2/3 -> Subsystem2/5(In5)
  Demux3/5 -> Subsystem4/6(In6)
  In5/1 -> Demux2/1
  Demux1/7 -> Subsystem6/4(In4)
  Subsystem7/1(Out1) -> Mux/8
  Demux/4 -> Subsystem3/3(In3)
  Demux2/1 -> Subsystem/5(In5)

== system cpu_von_nuemann/CPU/ALU/Subsystem7/Subsystem3/Subsystem1 ==
  In1 : Inport
  In2 : Inport  Port=2
  In3 : Inport  Port=3
  In4 : Inport  Port=4
  In5 : Inport  Port=5
  In7 : Inport  Port=6
  In6 : Inport  Port=7
  Demux{,1..3} (4 alike) : Demux  Outputs=8
  Mux : Mux  Inputs=8
  Subsystem : Subsystem
  Subsystem1 : Subsystem
  Subsystem2 : Subsystem
  Subsystem3 : Subsystem
  Subsystem4 : Subsystem
  Subsystem5 : Subsystem
  Subsystem6 : Subsystem
  Subsystem7 : Subsystem
  Out1 : Outport
  wires:
  Demux3/7 -> Subsystem6/6(In6)
  In6/1 -> Subsystem4/7(In7), Subsystem7/7(In7), Subsystem5/7(In7), Subsystem6/7(In7), Subsystem1/7(In7), Subsystem3/7(In7), Subsystem2/7(In7), Subsystem/7(In7)
  Subsystem3/1(Out1) -> Mux/4
  Demux/1 -> Subsystem/3(In3)
  Demux2/8 -> Subsystem7/5(In5)
  Subsystem1/1(Out1) -> Mux/2
  Subsystem2/1(Out1) -> Mux/3
  Subsystem4/1(Out1) -> Mux/5
  Demux1/2 -> Subsystem1/4(In4)
  Demux/6 -> Subsystem5/3(In3)
  In4/1 -> Demux1/1
  Demux2/7 -> Subsystem6/5(In5)
  In3/1 -> Demux/1
  Demux1/4 -> Subsystem3/4(In4)
  In2/1 -> Subsystem4/2(In2), Subsystem5/2(In2), Subsystem6/2(In2), Subsystem7/2(In2), Subsystem2/2(In2), Subsystem3/2(In2), Subsystem/2(In2), Subsystem1/2(In2)
  Demux3/3 -> Subsystem2/6(In6)
  Subsystem/1(Out1) -> Mux/1
  Subsystem5/1(Out1) -> Mux/6
  In7/1 -> Demux3/1
  Mux/1 -> Out1/1
  Demux/3 -> Subsystem2/3(In3)
  Demux1/8 -> Subsystem7/4(In4)
  Demux3/6 -> Subsystem5/6(In6)
  Demux3/1 -> Subsystem/6(In6)
  Demux3/2 -> Subsystem1/6(In6)
  Subsystem6/1(Out1) -> Mux/7
  Demux1/3 -> Subsystem2/4(In4)
  Demux2/4 -> Subsystem3/5(In5)
  Demux1/5 -> Subsystem4/4(In4)
  In1/1 -> Subsystem6/1(In1), Subsystem7/1(In1), Subsystem4/1(In1), Subsystem5/1(In1), Subsystem2/1(In1), Subsystem3/1(In1), Subsystem/1(In1), Subsystem1/1(In1)
  Demux1/1 -> Subsystem/4(In4)
  Demux3/4 -> Subsystem3/6(In6)
  Demux2/2 -> Subsystem1/5(In5)
  Demux2/6 -> Subsystem5/5(In5)
  Demux/2 -> Subsystem1/3(In3)
  Demux/7 -> Subsystem6/3(In3)
  Demux3/8 -> Subsystem7/6(In6)
  Demux1/6 -> Subsystem5/4(In4)
  Demux/5 -> Subsystem4/3(In3)
  Demux2/5 -> Subsystem4/5(In5)
  Demux/8 -> Subsystem7/3(In3)
  Demux2/3 -> Subsystem2/5(In5)
  Demux3/5 -> Subsystem4/6(In6)
  In5/1 -> Demux2/1
  Demux1/7 -> Subsystem6/4(In4)
  Subsystem7/1(Out1) -> Mux/8
  Demux/4 -> Subsystem3/3(In3)
  Demux2/1 -> Subsystem/5(In5)

== system cpu_von_nuemann/CPU/ALU/Subsystem7/Subsystem3/Subsystem2 ==
  In1 : Inport
  In2 : Inport  Port=2
  In3 : Inport  Port=3
  In4 : Inport  Port=4
  In5 : Inport  Port=5
  In7 : Inport  Port=6
  In6 : Inport  Port=7
  Demux{,1..3} (4 alike) : Demux  Outputs=8
  Mux : Mux  Inputs=8
  Subsystem : Subsystem
  Subsystem1 : Subsystem
  Subsystem2 : Subsystem
  Subsystem3 : Subsystem
  Subsystem4 : Subsystem
  Subsystem5 : Subsystem
  Subsystem6 : Subsystem
  Subsystem7 : Subsystem
  Out1 : Outport
  wires:
  Demux3/7 -> Subsystem6/6(In6)
  In6/1 -> Subsystem4/7(In7), Subsystem7/7(In7), Subsystem5/7(In7), Subsystem6/7(In7), Subsystem1/7(In7), Subsystem3/7(In7), Subsystem2/7(In7), Subsystem/7(In7)
  Subsystem3/1(Out1) -> Mux/4
  Demux/1 -> Subsystem/3(In3)
  Demux2/8 -> Subsystem7/5(In5)
  Subsystem1/1(Out1) -> Mux/2
  Subsystem2/1(Out1) -> Mux/3
  Subsystem4/1(Out1) -> Mux/5
  Demux1/2 -> Subsystem1/4(In4)
  Demux/6 -> Subsystem5/3(In3)
  In4/1 -> Demux1/1
  Demux2/7 -> Subsystem6/5(In5)
  In3/1 -> Demux/1
  Demux1/4 -> Subsystem3/4(In4)
  In2/1 -> Subsystem4/2(In2), Subsystem5/2(In2), Subsystem6/2(In2), Subsystem7/2(In2), Subsystem2/2(In2), Subsystem3/2(In2), Subsystem/2(In2), Subsystem1/2(In2)
  Demux3/3 -> Subsystem2/6(In6)
  Subsystem/1(Out1) -> Mux/1
  Subsystem5/1(Out1) -> Mux/6
  In7/1 -> Demux3/1
  Mux/1 -> Out1/1
  Demux/3 -> Subsystem2/3(In3)
  Demux1/8 -> Subsystem7/4(In4)
  Demux3/6 -> Subsystem5/6(In6)
  Demux3/1 -> Subsystem/6(In6)
  Demux3/2 -> Subsystem1/6(In6)
  Subsystem6/1(Out1) -> Mux/7
  Demux1/3 -> Subsystem2/4(In4)
  Demux2/4 -> Subsystem3/5(In5)
  Demux1/5 -> Subsystem4/4(In4)
  In1/1 -> Subsystem6/1(In1), Subsystem7/1(In1), Subsystem4/1(In1), Subsystem5/1(In1), Subsystem2/1(In1), Subsystem3/1(In1), Subsystem/1(In1), Subsystem1/1(In1)
  Demux1/1 -> Subsystem/4(In4)
  Demux3/4 -> Subsystem3/6(In6)
  Demux2/2 -> Subsystem1/5(In5)
  Demux2/6 -> Subsystem5/5(In5)
  Demux/2 -> Subsystem1/3(In3)
  Demux/7 -> Subsystem6/3(In3)
  Demux3/8 -> Subsystem7/6(In6)
  Demux1/6 -> Subsystem5/4(In4)
  Demux/5 -> Subsystem4/3(In3)
  Demux2/5 -> Subsystem4/5(In5)
  Demux/8 -> Subsystem7/3(In3)
  Demux2/3 -> Subsystem2/5(In5)
  Demux3/5 -> Subsystem4/6(In6)
  In5/1 -> Demux2/1
  Demux1/7 -> Subsystem6/4(In4)
  Subsystem7/1(Out1) -> Mux/8
  Demux/4 -> Subsystem3/3(In3)
  Demux2/1 -> Subsystem/5(In5)

== system cpu_von_nuemann/CPU/ALU/Subsystem7/Subsystem3/Subsystem3 ==
  In1 : Inport
  In2 : Inport  Port=2
  In3 : Inport  Port=3
  In4 : Inport  Port=4
  In5 : Inport  Port=5
  In7 : Inport  Port=6
  In6 : Inport  Port=7
  Demux{,1..3} (4 alike) : Demux  Outputs=8
  Mux : Mux  Inputs=8
  Subsystem : Subsystem
  Subsystem1 : Subsystem
  Subsystem2 : Subsystem
  Subsystem3 : Subsystem
  Subsystem4 : Subsystem
  Subsystem5 : Subsystem
  Subsystem6 : Subsystem
  Subsystem7 : Subsystem
  Out1 : Outport
  wires:
  Demux3/7 -> Subsystem6/6(In6)
  In6/1 -> Subsystem4/7(In7), Subsystem7/7(In7), Subsystem5/7(In7), Subsystem6/7(In7), Subsystem1/7(In7), Subsystem3/7(In7), Subsystem2/7(In7), Subsystem/7(In7)
  Subsystem3/1(Out1) -> Mux/4
  Demux/1 -> Subsystem/3(In3)
  Demux2/8 -> Subsystem7/5(In5)
  Subsystem1/1(Out1) -> Mux/2
  Subsystem2/1(Out1) -> Mux/3
  Subsystem4/1(Out1) -> Mux/5
  Demux1/2 -> Subsystem1/4(In4)
  Demux/6 -> Subsystem5/3(In3)
  In4/1 -> Demux1/1
  Demux2/7 -> Subsystem6/5(In5)
  In3/1 -> Demux/1
  Demux1/4 -> Subsystem3/4(In4)
  In2/1 -> Subsystem4/2(In2), Subsystem5/2(In2), Subsystem6/2(In2), Subsystem7/2(In2), Subsystem2/2(In2), Subsystem3/2(In2), Subsystem/2(In2), Subsystem1/2(In2)
  Demux3/3 -> Subsystem2/6(In6)
  Subsystem/1(Out1) -> Mux/1
  Subsystem5/1(Out1) -> Mux/6
  In7/1 -> Demux3/1
  Mux/1 -> Out1/1
  Demux/3 -> Subsystem2/3(In3)
  Demux1/8 -> Subsystem7/4(In4)
  Demux3/6 -> Subsystem5/6(In6)
  Demux3/1 -> Subsystem/6(In6)
  Demux3/2 -> Subsystem1/6(In6)
  Subsystem6/1(Out1) -> Mux/7
  Demux1/3 -> Subsystem2/4(In4)
  Demux2/4 -> Subsystem3/5(In5)
  Demux1/5 -> Subsystem4/4(In4)
  In1/1 -> Subsystem6/1(In1), Subsystem7/1(In1), Subsystem4/1(In1), Subsystem5/1(In1), Subsystem2/1(In1), Subsystem3/1(In1), Subsystem/1(In1), Subsystem1/1(In1)
  Demux1/1 -> Subsystem/4(In4)
  Demux3/4 -> Subsystem3/6(In6)
  Demux2/2 -> Subsystem1/5(In5)
  Demux2/6 -> Subsystem5/5(In5)
  Demux/2 -> Subsystem1/3(In3)
  Demux/7 -> Subsystem6/3(In3)
  Demux3/8 -> Subsystem7/6(In6)
  Demux1/6 -> Subsystem5/4(In4)
  Demux/5 -> Subsystem4/3(In3)
  Demux2/5 -> Subsystem4/5(In5)
  Demux/8 -> Subsystem7/3(In3)
  Demux2/3 -> Subsystem2/5(In5)
  Demux3/5 -> Subsystem4/6(In6)
  In5/1 -> Demux2/1
  Demux1/7 -> Subsystem6/4(In4)
  Subsystem7/1(Out1) -> Mux/8
  Demux/4 -> Subsystem3/3(In3)
  Demux2/1 -> Subsystem/5(In5)

== system cpu_von_nuemann/CPU/ALU/Subsystem7/Subsystem3/Subsystem4 ==
  In1 : Inport
  In2 : Inport  Port=2
  In3 : Inport  Port=3
  In4 : Inport  Port=4
  In5 : Inport  Port=5
  In7 : Inport  Port=6
  In6 : Inport  Port=7
  Demux{,1..3} (4 alike) : Demux  Outputs=8
  Mux : Mux  Inputs=8
  Subsystem : Subsystem
  Subsystem1 : Subsystem
  Subsystem2 : Subsystem
  Subsystem3 : Subsystem
  Subsystem4 : Subsystem
  Subsystem5 : Subsystem
  Subsystem6 : Subsystem
  Subsystem7 : Subsystem
  Out1 : Outport
  wires:
  Demux3/7 -> Subsystem6/6(In6)
  In6/1 -> Subsystem4/7(In7), Subsystem7/7(In7), Subsystem5/7(In7), Subsystem6/7(In7), Subsystem1/7(In7), Subsystem3/7(In7), Subsystem2/7(In7), Subsystem/7(In7)
  Subsystem3/1(Out1) -> Mux/4
  Demux/1 -> Subsystem/3(In3)
  Demux2/8 -> Subsystem7/5(In5)
  Subsystem1/1(Out1) -> Mux/2
  Subsystem2/1(Out1) -> Mux/3
  Subsystem4/1(Out1) -> Mux/5
  Demux1/2 -> Subsystem1/4(In4)
  Demux/6 -> Subsystem5/3(In3)
  In4/1 -> Demux1/1
  Demux2/7 -> Subsystem6/5(In5)
  In3/1 -> Demux/1
  Demux1/4 -> Subsystem3/4(In4)
  In2/1 -> Subsystem4/2(In2), Subsystem5/2(In2), Subsystem6/2(In2), Subsystem7/2(In2), Subsystem2/2(In2), Subsystem3/2(In2), Subsystem/2(In2), Subsystem1/2(In2)
  Demux3/3 -> Subsystem2/6(In6)
  Subsystem/1(Out1) -> Mux/1
  Subsystem5/1(Out1) -> Mux/6
  In7/1 -> Demux3/1
  Mux/1 -> Out1/1
  Demux/3 -> Subsystem2/3(In3)
  Demux1/8 -> Subsystem7/4(In4)
  Demux3/6 -> Subsystem5/6(In6)
  Demux3/1 -> Subsystem/6(In6)
  Demux3/2 -> Subsystem1/6(In6)
  Subsystem6/1(Out1) -> Mux/7
  Demux1/3 -> Subsystem2/4(In4)
  Demux2/4 -> Subsystem3/5(In5)
  Demux1/5 -> Subsystem4/4(In4)
  In1/1 -> Subsystem6/1(In1), Subsystem7/1(In1), Subsystem4/1(In1), Subsystem5/1(In1), Subsystem2/1(In1), Subsystem3/1(In1), Subsystem/1(In1), Subsystem1/1(In1)
  Demux1/1 -> Subsystem/4(In4)
  Demux3/4 -> Subsystem3/6(In6)
  Demux2/2 -> Subsystem1/5(In5)
  Demux2/6 -> Subsystem5/5(In5)
  Demux/2 -> Subsystem1/3(In3)
  Demux/7 -> Subsystem6/3(In3)
  Demux3/8 -> Subsystem7/6(In6)
  Demux1/6 -> Subsystem5/4(In4)
  Demux/5 -> Subsystem4/3(In3)
  Demux2/5 -> Subsystem4/5(In5)
  Demux/8 -> Subsystem7/3(In3)
  Demux2/3 -> Subsystem2/5(In5)
  Demux3/5 -> Subsystem4/6(In6)
  In5/1 -> Demux2/1
  Demux1/7 -> Subsystem6/4(In4)
  Subsystem7/1(Out1) -> Mux/8
  Demux/4 -> Subsystem3/3(In3)
  Demux2/1 -> Subsystem/5(In5)

== system cpu_von_nuemann/CPU/ALU/Subsystem7/Subsystem3/Subsystem5 ==
  In1 : Inport
  In2 : Inport  Port=2
  In3 : Inport  Port=3
  In4 : Inport  Port=4
  In5 : Inport  Port=5
  In7 : Inport  Port=6
  In6 : Inport  Port=7
  Demux{,1..3} (4 alike) : Demux  Outputs=8
  Mux : Mux  Inputs=8
  Subsystem : Subsystem
  Subsystem1 : Subsystem
  Subsystem2 : Subsystem
  Subsystem3 : Subsystem
  Subsystem4 : Subsystem
  Subsystem5 : Subsystem
  Subsystem6 : Subsystem
  Subsystem7 : Subsystem
  Out1 : Outport
  wires:
  Demux3/7 -> Subsystem6/6(In6)
  In6/1 -> Subsystem4/7(In7), Subsystem7/7(In7), Subsystem5/7(In7), Subsystem6/7(In7), Subsystem1/7(In7), Subsystem3/7(In7), Subsystem2/7(In7), Subsystem/7(In7)
  Subsystem3/1(Out1) -> Mux/4
  Demux/1 -> Subsystem/3(In3)
  Demux2/8 -> Subsystem7/5(In5)
  Subsystem1/1(Out1) -> Mux/2
  Subsystem2/1(Out1) -> Mux/3
  Subsystem4/1(Out1) -> Mux/5
  Demux1/2 -> Subsystem1/4(In4)
  Demux/6 -> Subsystem5/3(In3)
  In4/1 -> Demux1/1
  Demux2/7 -> Subsystem6/5(In5)
  In3/1 -> Demux/1
  Demux1/4 -> Subsystem3/4(In4)
  In2/1 -> Subsystem4/2(In2), Subsystem5/2(In2), Subsystem6/2(In2), Subsystem7/2(In2), Subsystem2/2(In2), Subsystem3/2(In2), Subsystem/2(In2), Subsystem1/2(In2)
  Demux3/3 -> Subsystem2/6(In6)
  Subsystem/1(Out1) -> Mux/1
  Subsystem5/1(Out1) -> Mux/6
  In7/1 -> Demux3/1
  Mux/1 -> Out1/1
  Demux/3 -> Subsystem2/3(In3)
  Demux1/8 -> Subsystem7/4(In4)
  Demux3/6 -> Subsystem5/6(In6)
  Demux3/1 -> Subsystem/6(In6)
  Demux3/2 -> Subsystem1/6(In6)
  Subsystem6/1(Out1) -> Mux/7
  Demux1/3 -> Subsystem2/4(In4)
  Demux2/4 -> Subsystem3/5(In5)
  Demux1/5 -> Subsystem4/4(In4)
  In1/1 -> Subsystem6/1(In1), Subsystem7/1(In1), Subsystem4/1(In1), Subsystem5/1(In1), Subsystem2/1(In1), Subsystem3/1(In1), Subsystem/1(In1), Subsystem1/1(In1)
  Demux1/1 -> Subsystem/4(In4)
  Demux3/4 -> Subsystem3/6(In6)
  Demux2/2 -> Subsystem1/5(In5)
  Demux2/6 -> Subsystem5/5(In5)
  Demux/2 -> Subsystem1/3(In3)
  Demux/7 -> Subsystem6/3(In3)
  Demux3/8 -> Subsystem7/6(In6)
  Demux1/6 -> Subsystem5/4(In4)
  Demux/5 -> Subsystem4/3(In3)
  Demux2/5 -> Subsystem4/5(In5)
  Demux/8 -> Subsystem7/3(In3)
  Demux2/3 -> Subsystem2/5(In5)
  Demux3/5 -> Subsystem4/6(In6)
  In5/1 -> Demux2/1
  Demux1/7 -> Subsystem6/4(In4)
  Subsystem7/1(Out1) -> Mux/8
  Demux/4 -> Subsystem3/3(In3)
  Demux2/1 -> Subsystem/5(In5)

== system cpu_von_nuemann/CPU/ALU/Subsystem7/Subsystem4/Subsystem1 ==
  In1 : Inport
  In2 : Inport  Port=2
  In3 : Inport  Port=3
  In4 : Inport  Port=4
  In5 : Inport  Port=5
  In7 : Inport  Port=6
  In6 : Inport  Port=7
  Demux{,1..3} (4 alike) : Demux  Outputs=8
  Mux : Mux  Inputs=8
  Subsystem : Subsystem
  Subsystem1 : Subsystem
  Subsystem2 : Subsystem
  Subsystem3 : Subsystem
  Subsystem4 : Subsystem
  Subsystem5 : Subsystem
  Subsystem6 : Subsystem
  Subsystem7 : Subsystem
  Out1 : Outport
  wires:
  Demux3/7 -> Subsystem6/6(In6)
  In6/1 -> Subsystem4/7(In7), Subsystem7/7(In7), Subsystem5/7(In7), Subsystem6/7(In7), Subsystem1/7(In7), Subsystem3/7(In7), Subsystem2/7(In7), Subsystem/7(In7)
  Subsystem3/1(Out1) -> Mux/4
  Demux/1 -> Subsystem/3(In3)
  Demux2/8 -> Subsystem7/5(In5)
  Subsystem1/1(Out1) -> Mux/2
  Subsystem2/1(Out1) -> Mux/3
  Subsystem4/1(Out1) -> Mux/5
  Demux1/2 -> Subsystem1/4(In4)
  Demux/6 -> Subsystem5/3(In3)
  In4/1 -> Demux1/1
  Demux2/7 -> Subsystem6/5(In5)
  In3/1 -> Demux/1
  Demux1/4 -> Subsystem3/4(In4)
  In2/1 -> Subsystem4/2(In2), Subsystem5/2(In2), Subsystem6/2(In2), Subsystem7/2(In2), Subsystem2/2(In2), Subsystem3/2(In2), Subsystem/2(In2), Subsystem1/2(In2)
  Demux3/3 -> Subsystem2/6(In6)
  Subsystem/1(Out1) -> Mux/1
  Subsystem5/1(Out1) -> Mux/6
  In7/1 -> Demux3/1
  Mux/1 -> Out1/1
  Demux/3 -> Subsystem2/3(In3)
  Demux1/8 -> Subsystem7/4(In4)
  Demux3/6 -> Subsystem5/6(In6)
  Demux3/1 -> Subsystem/6(In6)
  Demux3/2 -> Subsystem1/6(In6)
  Subsystem6/1(Out1) -> Mux/7
  Demux1/3 -> Subsystem2/4(In4)
  Demux2/4 -> Subsystem3/5(In5)
  Demux1/5 -> Subsystem4/4(In4)
  In1/1 -> Subsystem6/1(In1), Subsystem7/1(In1), Subsystem4/1(In1), Subsystem5/1(In1), Subsystem2/1(In1), Subsystem3/1(In1), Subsystem/1(In1), Subsystem1/1(In1)
  Demux1/1 -> Subsystem/4(In4)
  Demux3/4 -> Subsystem3/6(In6)
  Demux2/2 -> Subsystem1/5(In5)
  Demux2/6 -> Subsystem5/5(In5)
  Demux/2 -> Subsystem1/3(In3)
  Demux/7 -> Subsystem6/3(In3)
  Demux3/8 -> Subsystem7/6(In6)
  Demux1/6 -> Subsystem5/4(In4)
  Demux/5 -> Subsystem4/3(In3)
  Demux2/5 -> Subsystem4/5(In5)
  Demux/8 -> Subsystem7/3(In3)
  Demux2/3 -> Subsystem2/5(In5)
  Demux3/5 -> Subsystem4/6(In6)
  In5/1 -> Demux2/1
  Demux1/7 -> Subsystem6/4(In4)
  Subsystem7/1(Out1) -> Mux/8
  Demux/4 -> Subsystem3/3(In3)
  Demux2/1 -> Subsystem/5(In5)
